simulink library "dsrc_transmitter"  (Simulink 8.2)
settings: Solver=ode1  StartTime=0.0  StopTime=Inf  FixedStep=0.001  RelTol=1e-3
PostLoadFcn:
  | , if any(exist('dsrtsu_mdlpostloadfcn', 'file') == [2, 3, 6]), try dsrtsu_mdlpostloadfcn('Execute', bdroot); catch fprintf('Error in PostLoadFcn (dsrtsu_mdlpostloadfcn) for model "%s":\n %s\n', bdroot, lasterr); end, end,
libraries: simulink x10, rtitttasklib x2, rtiethernetudplib x1, parse_utils x1
(part 2 of 2)

== system dsrc_transmitter/BSM Broadcast/Write TORC Data/Veh 3 Data Update ==
  BSM Data1 : Inport
  Action Port : ActionPort
  Bus Selector : BusSelector  OutputSignals=signal1 (signal 1),value (signal 2),value (signal 3),signal4 (signal 4),signal5 (signal 5),signal6 (signal 6),value (signal 7),value (signal 8),value (signal 9),value (signal 10),value (signal 11),value (signal 12),value (signal 13),value (signal 14),value (signal 15),signal16 (signal 16),signal17 (signal 17),signal18 (signal 18),signal19 (signal 19),signal20 (signal 20),signal21 (signal 21),signal22 (signal 22),signal23 (signal 23),signal24 (signal 24),signal25 (signal 25),value (signal 26),value (signal 27),signal28 (signal 28),value (signal 29),signal30 (signal 30),value (signal 31),signal32 (signal 32),signal33 (signal 33),value (signal 34),value (signal 35),signal36 (signal 36),signal37 (signal 37),signal38 (signal 38),signal39 (signal 39),signal40 (signal 40),signal41 (signal 41),signal42 (signal 42),signal43 (signal 43),signal44 (signal 44),signal45 (signal 45)
  Data Store Write1 : DataStoreWrite  DataStoreName=BSMStoreSignal  DataStoreElements=BSMStoreSignal.Veh3BSM.caccFlags_bitmask#BSMStoreSignal.Veh3BSM.setSpeed_m_s#BSMStoreSignal.Veh3BSM.throtPos_percent#BSMStoreSignal.Veh3BSM.lclPN_mm#BSMStoreSignal.Veh3BSM.lclPE_mm#BSMStoreSignal.Veh3BSM.lclPD_mm#BSMStoreSignal.Veh3BSM.roll_deg#BSMStoreSignal.Veh3BSM.pitch_deg#BSMStoreSignal.Veh3BSM.yaw_deg#BSMStoreSignal.Veh3BSM.hPosAcry_m#BSMStoreSignal.Veh3BSM.vPosAcry_m#BSMStoreSignal.Veh3BSM.frwdVel_m_s#BSMStoreSignal.Veh3BSM.rightVel_m_s#BSMStoreSignal.Veh3BSM.downVel_m_s#BSMStoreSignal.Veh3BSM.velAcc_m_s#BSMStoreSignal.Veh3BSM.frwdAcc_mm_s_s#BSMStoreSignal.Veh3BSM.rightAcc_mm_s_s#BSMStoreSignal.Veh3BSM.dwnAcc_mm_s_s#BSMStoreSignal.Veh3BSM.msgID#BSMStoreSignal.Veh3BSM.msgCnt#BSMStoreSignal.Veh3BSM.id#BSMStoreSignal.Veh3BSM.secMark_ms#BSMStoreSignal.Veh3BSM.lat_deg#BSMStoreSignal.Veh3BSM.lon_deg#BSMStoreSignal.Veh3BSM.elev_m#BSMStoreSignal.Veh3BSM.semi_major_accuracy_m#BSMStoreSignal.Veh3BSM.semi_minor_accuracy_m#BSMStoreSignal.Veh3BSM.semi_major_accuracy_orientation_deg#BSMStoreSignal.Veh3BSM.speed_m_s#BSMStoreSignal.Veh3BSM.transmission_enum#BSMStoreSignal.Veh3BSM.heading_deg#BSMStoreSignal.Veh3BSM.angle_deg#BSMStoreSignal.Veh3BSM.vertical_acceleration_g#BSMStoreSignal.Veh3BSM.lat_acceleration_m_s_s#BSMStoreSignal.Veh3BSM.long_acceleration_m_s_s#BSMStoreSignal.Veh3BSM.yaw_rate_deg_s#BSMStoreSignal.Veh3BSM.wheelBrakes_bitmask#BSMStoreSignal.Veh3BSM.wheelBrakesUnavailable#BSMStoreSignal.Veh3BSM.tractionControlState_enum#BSMStoreSignal.Veh3BSM.anti_lock_brake_status_enum#BSMStoreSignal.Veh3BSM.stability_control_status_enum#BSMStoreSignal.Veh3BSM.brake_boost_enum#BSMStoreSignal.Veh3BSM.auxiliary_brakes_status_enum#BSMStoreSignal.Veh3BSM.vehicle_height_cm#BSMStoreSignal.Veh3BSM.vehicle_width_cm
  wires:
  BSM Data1/1 -> Bus Selector/1
  Bus Selector/31 -> Data Store Write1/31  "<value (signal 31)>"
  Bus Selector/10 -> Data Store Write1/10  "<value (signal 10)>"
  Bus Selector/8 -> Data Store Write1/8  "<value (signal 8)>"
  Bus Selector/13 -> Data Store Write1/13  "<value (signal 13)>"
  Bus Selector/11 -> Data Store Write1/11  "<value (signal 11)>"
  Bus Selector/12 -> Data Store Write1/12  "<value (signal 12)>"
  Bus Selector/19 -> Data Store Write1/19  "<signal19 (signal 19)>"
  Bus Selector/20 -> Data Store Write1/20  "<signal20 (signal 20)>"
  Bus Selector/18 -> Data Store Write1/18  "<signal18 (signal 18)>"
  Bus Selector/14 -> Data Store Write1/14  "<value (signal 14)>"
  Bus Selector/22 -> Data Store Write1/22  "<signal22 (signal 22)>"
  Bus Selector/44 -> Data Store Write1/44  "<signal44 (signal 44)>"
  Bus Selector/42 -> Data Store Write1/42  "<signal42 (signal 42)>"
  Bus Selector/35 -> Data Store Write1/35  "<value (signal 35)>"
  Bus Selector/36 -> Data Store Write1/36  "<signal36 (signal 36)>"
  Bus Selector/45 -> Data Store Write1/45  "<signal45 (signal 45)>"
  Bus Selector/7 -> Data Store Write1/7  "<value (signal 7)>"
  Bus Selector/39 -> Data Store Write1/39  "<signal39 (signal 39)>"
  Bus Selector/23 -> Data Store Write1/23  "<signal23 (signal 23)>"
  Bus Selector/43 -> Data Store Write1/43  "<signal43 (signal 43)>"
  Bus Selector/28 -> Data Store Write1/28  "<signal28 (signal 28)>"
  Bus Selector/29 -> Data Store Write1/29  "<value (signal 29)>"
  Bus Selector/25 -> Data Store Write1/25  "<signal25 (signal 25)>"
  Bus Selector/30 -> Data Store Write1/30  "<signal30 (signal 30)>"
  Bus Selector/32 -> Data Store Write1/32  "<signal32 (signal 32)>"
  Bus Selector/27 -> Data Store Write1/27  "<value (signal 27)>"
  Bus Selector/26 -> Data Store Write1/26  "<value (signal 26)>"
  Bus Selector/24 -> Data Store Write1/24  "<signal24 (signal 24)>"
  Bus Selector/16 -> Data Store Write1/16  "<signal16 (signal 16)>"
  Bus Selector/33 -> Data Store Write1/33  "<signal33 (signal 33)>"
  Bus Selector/17 -> Data Store Write1/17  "<signal17 (signal 17)>"
  Bus Selector/15 -> Data Store Write1/15  "<value (signal 15)>"
  Bus Selector/41 -> Data Store Write1/41  "<signal41 (signal 41)>"
  Bus Selector/37 -> Data Store Write1/37  "<signal37 (signal 37)>"
  Bus Selector/9 -> Data Store Write1/9  "<value (signal 9)>"
  Bus Selector/3 -> Data Store Write1/3  "<value (signal 3)>"
  Bus Selector/38 -> Data Store Write1/38  "<signal38 (signal 38)>"
  Bus Selector/5 -> Data Store Write1/5  "<signal5 (signal 5)>"
  Bus Selector/4 -> Data Store Write1/4  "<signal4 (signal 4)>"
  Bus Selector/1 -> Data Store Write1/1  "<signal1 (signal 1)>"
  Bus Selector/40 -> Data Store Write1/40  "<signal40 (signal 40)>"
  Bus Selector/2 -> Data Store Write1/2  "<value (signal 2)>"
  Bus Selector/34 -> Data Store Write1/34  "<value (signal 34)>"
  Bus Selector/21 -> Data Store Write1/21  "<signal21 (signal 21)>"
  Bus Selector/6 -> Data Store Write1/6  "<signal6 (signal 6)>"

== system dsrc_transmitter/BSM Broadcast/Write TORC Data/Veh 4 Data Update ==
  BSM Data : Inport
  Action Port : ActionPort
  Bus Selector : BusSelector  OutputSignals=signal1 (signal 1),value (signal 2),value (signal 3),signal4 (signal 4),signal5 (signal 5),signal6 (signal 6),value (signal 7),value (signal 8),value (signal 9),value (signal 10),value (signal 11),value (signal 12),value (signal 13),value (signal 14),value (signal 15),signal16 (signal 16),signal17 (signal 17),signal18 (signal 18),signal19 (signal 19),signal20 (signal 20),signal21 (signal 21),signal22 (signal 22),signal23 (signal 23),signal24 (signal 24),signal25 (signal 25),value (signal 26),value (signal 27),signal28 (signal 28),value (signal 29),signal30 (signal 30),value (signal 31),signal32 (signal 32),signal33 (signal 33),value (signal 34),value (signal 35),signal36 (signal 36),signal37 (signal 37),signal38 (signal 38),signal39 (signal 39),signal40 (signal 40),signal41 (signal 41),signal42 (signal 42),signal43 (signal 43),signal44 (signal 44),signal45 (signal 45)
  Data Store Write1 : DataStoreWrite  DataStoreName=BSMStoreSignal  DataStoreElements=BSMStoreSignal.Veh4BSM.caccFlags_bitmask#BSMStoreSignal.Veh4BSM.setSpeed_m_s#BSMStoreSignal.Veh4BSM.throtPos_percent#BSMStoreSignal.Veh4BSM.lclPN_mm#BSMStoreSignal.Veh4BSM.lclPE_mm#BSMStoreSignal.Veh4BSM.lclPD_mm#BSMStoreSignal.Veh4BSM.roll_deg#BSMStoreSignal.Veh4BSM.pitch_deg#BSMStoreSignal.Veh4BSM.yaw_deg#BSMStoreSignal.Veh4BSM.hPosAcry_m#BSMStoreSignal.Veh4BSM.vPosAcry_m#BSMStoreSignal.Veh4BSM.frwdVel_m_s#BSMStoreSignal.Veh4BSM.rightVel_m_s#BSMStoreSignal.Veh4BSM.downVel_m_s#BSMStoreSignal.Veh4BSM.velAcc_m_s#BSMStoreSignal.Veh4BSM.frwdAcc_mm_s_s#BSMStoreSignal.Veh4BSM.rightAcc_mm_s_s#BSMStoreSignal.Veh4BSM.dwnAcc_mm_s_s#BSMStoreSignal.Veh4BSM.msgID#BSMStoreSignal.Veh4BSM.msgCnt#BSMStoreSignal.Veh4BSM.id#BSMStoreSignal.Veh4BSM.secMark_ms#BSMStoreSignal.Veh4BSM.lat_deg#BSMStoreSignal.Veh4BSM.lon_deg#BSMStoreSignal.Veh4BSM.elev_m#BSMStoreSignal.Veh4BSM.semi_major_accuracy_m#BSMStoreSignal.Veh4BSM.semi_minor_accuracy_m#BSMStoreSignal.Veh4BSM.semi_major_accuracy_orientation_deg#BSMStoreSignal.Veh4BSM.speed_m_s#BSMStoreSignal.Veh4BSM.transmission_enum#BSMStoreSignal.Veh4BSM.heading_deg#BSMStoreSignal.Veh4BSM.angle_deg#BSMStoreSignal.Veh4BSM.vertical_acceleration_g#BSMStoreSignal.Veh4BSM.lat_acceleration_m_s_s#BSMStoreSignal.Veh4BSM.long_acceleration_m_s_s#BSMStoreSignal.Veh4BSM.yaw_rate_deg_s#BSMStoreSignal.Veh4BSM.wheelBrakes_bitmask#BSMStoreSignal.Veh4BSM.wheelBrakesUnavailable#BSMStoreSignal.Veh4BSM.tractionControlState_enum#BSMStoreSignal.Veh4BSM.anti_lock_brake_status_enum#BSMStoreSignal.Veh4BSM.stability_control_status_enum#BSMStoreSignal.Veh4BSM.brake_boost_enum#BSMStoreSignal.Veh4BSM.auxiliary_brakes_status_enum#BSMStoreSignal.Veh4BSM.vehicle_height_cm#BSMStoreSignal.Veh4BSM.vehicle_width_cm
  wires:
  BSM Data/1 -> Bus Selector/1
  Bus Selector/31 -> Data Store Write1/31  "<value (signal 31)>"
  Bus Selector/10 -> Data Store Write1/10  "<value (signal 10)>"
  Bus Selector/8 -> Data Store Write1/8  "<value (signal 8)>"
  Bus Selector/13 -> Data Store Write1/13  "<value (signal 13)>"
  Bus Selector/11 -> Data Store Write1/11  "<value (signal 11)>"
  Bus Selector/12 -> Data Store Write1/12  "<value (signal 12)>"
  Bus Selector/19 -> Data Store Write1/19  "<signal19 (signal 19)>"
  Bus Selector/20 -> Data Store Write1/20  "<signal20 (signal 20)>"
  Bus Selector/18 -> Data Store Write1/18  "<signal18 (signal 18)>"
  Bus Selector/14 -> Data Store Write1/14  "<value (signal 14)>"
  Bus Selector/22 -> Data Store Write1/22  "<signal22 (signal 22)>"
  Bus Selector/44 -> Data Store Write1/44  "<signal44 (signal 44)>"
  Bus Selector/42 -> Data Store Write1/42  "<signal42 (signal 42)>"
  Bus Selector/35 -> Data Store Write1/35  "<value (signal 35)>"
  Bus Selector/36 -> Data Store Write1/36  "<signal36 (signal 36)>"
  Bus Selector/45 -> Data Store Write1/45  "<signal45 (signal 45)>"
  Bus Selector/7 -> Data Store Write1/7  "<value (signal 7)>"
  Bus Selector/39 -> Data Store Write1/39  "<signal39 (signal 39)>"
  Bus Selector/23 -> Data Store Write1/23  "<signal23 (signal 23)>"
  Bus Selector/43 -> Data Store Write1/43  "<signal43 (signal 43)>"
  Bus Selector/28 -> Data Store Write1/28  "<signal28 (signal 28)>"
  Bus Selector/29 -> Data Store Write1/29  "<value (signal 29)>"
  Bus Selector/25 -> Data Store Write1/25  "<signal25 (signal 25)>"
  Bus Selector/30 -> Data Store Write1/30  "<signal30 (signal 30)>"
  Bus Selector/32 -> Data Store Write1/32  "<signal32 (signal 32)>"
  Bus Selector/27 -> Data Store Write1/27  "<value (signal 27)>"
  Bus Selector/26 -> Data Store Write1/26  "<value (signal 26)>"
  Bus Selector/24 -> Data Store Write1/24  "<signal24 (signal 24)>"
  Bus Selector/16 -> Data Store Write1/16  "<signal16 (signal 16)>"
  Bus Selector/33 -> Data Store Write1/33  "<signal33 (signal 33)>"
  Bus Selector/17 -> Data Store Write1/17  "<signal17 (signal 17)>"
  Bus Selector/15 -> Data Store Write1/15  "<value (signal 15)>"
  Bus Selector/41 -> Data Store Write1/41  "<signal41 (signal 41)>"
  Bus Selector/37 -> Data Store Write1/37  "<signal37 (signal 37)>"
  Bus Selector/9 -> Data Store Write1/9  "<value (signal 9)>"
  Bus Selector/3 -> Data Store Write1/3  "<value (signal 3)>"
  Bus Selector/38 -> Data Store Write1/38  "<signal38 (signal 38)>"
  Bus Selector/5 -> Data Store Write1/5  "<signal5 (signal 5)>"
  Bus Selector/4 -> Data Store Write1/4  "<signal4 (signal 4)>"
  Bus Selector/1 -> Data Store Write1/1  "<signal1 (signal 1)>"
  Bus Selector/40 -> Data Store Write1/40  "<signal40 (signal 40)>"
  Bus Selector/2 -> Data Store Write1/2  "<value (signal 2)>"
  Bus Selector/34 -> Data Store Write1/34  "<value (signal 34)>"
  Bus Selector/21 -> Data Store Write1/21  "<signal21 (signal 21)>"
  Bus Selector/6 -> Data Store Write1/6  "<signal6 (signal 6)>"

== system dsrc_transmitter/BSM Broadcast/Write TORC Data/Veh 5 Data Update ==
  BSM Data : Inport
  Action Port : ActionPort
  Bus Selector : BusSelector  OutputSignals=signal1 (signal 1),value (signal 2),value (signal 3),signal4 (signal 4),signal5 (signal 5),signal6 (signal 6),value (signal 7),value (signal 8),value (signal 9),value (signal 10),value (signal 11),value (signal 12),value (signal 13),value (signal 14),value (signal 15),signal16 (signal 16),signal17 (signal 17),signal18 (signal 18),signal19 (signal 19),signal20 (signal 20),signal21 (signal 21),signal22 (signal 22),signal23 (signal 23),signal24 (signal 24),signal25 (signal 25),value (signal 26),value (signal 27),signal28 (signal 28),value (signal 29),signal30 (signal 30),value (signal 31),signal32 (signal 32),signal33 (signal 33),value (signal 34),value (signal 35),signal36 (signal 36),signal37 (signal 37),signal38 (signal 38),signal39 (signal 39),signal40 (signal 40),signal41 (signal 41),signal42 (signal 42),signal43 (signal 43),signal44 (signal 44),signal45 (signal 45)
  Data Store Write1 : DataStoreWrite  DataStoreName=BSMStoreSignal  DataStoreElements=BSMStoreSignal.Veh5BSM.caccFlags_bitmask#BSMStoreSignal.Veh5BSM.setSpeed_m_s#BSMStoreSignal.Veh5BSM.throtPos_percent#BSMStoreSignal.Veh5BSM.lclPN_mm#BSMStoreSignal.Veh5BSM.lclPE_mm#BSMStoreSignal.Veh5BSM.lclPD_mm#BSMStoreSignal.Veh5BSM.roll_deg#BSMStoreSignal.Veh5BSM.pitch_deg#BSMStoreSignal.Veh5BSM.yaw_deg#BSMStoreSignal.Veh5BSM.hPosAcry_m#BSMStoreSignal.Veh5BSM.vPosAcry_m#BSMStoreSignal.Veh5BSM.frwdVel_m_s#BSMStoreSignal.Veh5BSM.rightVel_m_s#BSMStoreSignal.Veh5BSM.downVel_m_s#BSMStoreSignal.Veh5BSM.velAcc_m_s#BSMStoreSignal.Veh5BSM.frwdAcc_mm_s_s#BSMStoreSignal.Veh5BSM.rightAcc_mm_s_s#BSMStoreSignal.Veh5BSM.dwnAcc_mm_s_s#BSMStoreSignal.Veh5BSM.msgID#BSMStoreSignal.Veh5BSM.msgCnt#BSMStoreSignal.Veh5BSM.id#BSMStoreSignal.Veh5BSM.secMark_ms#BSMStoreSignal.Veh5BSM.lat_deg#BSMStoreSignal.Veh5BSM.lon_deg#BSMStoreSignal.Veh5BSM.elev_m#BSMStoreSignal.Veh5BSM.semi_major_accuracy_m#BSMStoreSignal.Veh5BSM.semi_minor_accuracy_m#BSMStoreSignal.Veh5BSM.semi_major_accuracy_orientation_deg#BSMStoreSignal.Veh5BSM.speed_m_s#BSMStoreSignal.Veh5BSM.transmission_enum#BSMStoreSignal.Veh5BSM.heading_deg#BSMStoreSignal.Veh5BSM.angle_deg#BSMStoreSignal.Veh5BSM.vertical_acceleration_g#BSMStoreSignal.Veh5BSM.lat_acceleration_m_s_s#BSMStoreSignal.Veh5BSM.long_acceleration_m_s_s#BSMStoreSignal.Veh5BSM.yaw_rate_deg_s#BSMStoreSignal.Veh5BSM.wheelBrakes_bitmask#BSMStoreSignal.Veh5BSM.wheelBrakesUnavailable#BSMStoreSignal.Veh5BSM.tractionControlState_enum#BSMStoreSignal.Veh5BSM.anti_lock_brake_status_enum#BSMStoreSignal.Veh5BSM.stability_control_status_enum#BSMStoreSignal.Veh5BSM.brake_boost_enum#BSMStoreSignal.Veh5BSM.auxiliary_brakes_status_enum#BSMStoreSignal.Veh5BSM.vehicle_height_cm#BSMStoreSignal.Veh5BSM.vehicle_width_cm
  wires:
  BSM Data/1 -> Bus Selector/1
  Bus Selector/31 -> Data Store Write1/31  "<value (signal 31)>"
  Bus Selector/10 -> Data Store Write1/10  "<value (signal 10)>"
  Bus Selector/8 -> Data Store Write1/8  "<value (signal 8)>"
  Bus Selector/13 -> Data Store Write1/13  "<value (signal 13)>"
  Bus Selector/11 -> Data Store Write1/11  "<value (signal 11)>"
  Bus Selector/12 -> Data Store Write1/12  "<value (signal 12)>"
  Bus Selector/19 -> Data Store Write1/19  "<signal19 (signal 19)>"
  Bus Selector/20 -> Data Store Write1/20  "<signal20 (signal 20)>"
  Bus Selector/18 -> Data Store Write1/18  "<signal18 (signal 18)>"
  Bus Selector/14 -> Data Store Write1/14  "<value (signal 14)>"
  Bus Selector/22 -> Data Store Write1/22  "<signal22 (signal 22)>"
  Bus Selector/44 -> Data Store Write1/44  "<signal44 (signal 44)>"
  Bus Selector/42 -> Data Store Write1/42  "<signal42 (signal 42)>"
  Bus Selector/35 -> Data Store Write1/35  "<value (signal 35)>"
  Bus Selector/36 -> Data Store Write1/36  "<signal36 (signal 36)>"
  Bus Selector/45 -> Data Store Write1/45  "<signal45 (signal 45)>"
  Bus Selector/7 -> Data Store Write1/7  "<value (signal 7)>"
  Bus Selector/39 -> Data Store Write1/39  "<signal39 (signal 39)>"
  Bus Selector/23 -> Data Store Write1/23  "<signal23 (signal 23)>"
  Bus Selector/43 -> Data Store Write1/43  "<signal43 (signal 43)>"
  Bus Selector/28 -> Data Store Write1/28  "<signal28 (signal 28)>"
  Bus Selector/29 -> Data Store Write1/29  "<value (signal 29)>"
  Bus Selector/25 -> Data Store Write1/25  "<signal25 (signal 25)>"
  Bus Selector/30 -> Data Store Write1/30  "<signal30 (signal 30)>"
  Bus Selector/32 -> Data Store Write1/32  "<signal32 (signal 32)>"
  Bus Selector/27 -> Data Store Write1/27  "<value (signal 27)>"
  Bus Selector/26 -> Data Store Write1/26  "<value (signal 26)>"
  Bus Selector/24 -> Data Store Write1/24  "<signal24 (signal 24)>"
  Bus Selector/16 -> Data Store Write1/16  "<signal16 (signal 16)>"
  Bus Selector/33 -> Data Store Write1/33  "<signal33 (signal 33)>"
  Bus Selector/17 -> Data Store Write1/17  "<signal17 (signal 17)>"
  Bus Selector/15 -> Data Store Write1/15  "<value (signal 15)>"
  Bus Selector/41 -> Data Store Write1/41  "<signal41 (signal 41)>"
  Bus Selector/37 -> Data Store Write1/37  "<signal37 (signal 37)>"
  Bus Selector/9 -> Data Store Write1/9  "<value (signal 9)>"
  Bus Selector/3 -> Data Store Write1/3  "<value (signal 3)>"
  Bus Selector/38 -> Data Store Write1/38  "<signal38 (signal 38)>"
  Bus Selector/5 -> Data Store Write1/5  "<signal5 (signal 5)>"
  Bus Selector/4 -> Data Store Write1/4  "<signal4 (signal 4)>"
  Bus Selector/1 -> Data Store Write1/1  "<signal1 (signal 1)>"
  Bus Selector/40 -> Data Store Write1/40  "<signal40 (signal 40)>"
  Bus Selector/2 -> Data Store Write1/2  "<value (signal 2)>"
  Bus Selector/34 -> Data Store Write1/34  "<value (signal 34)>"
  Bus Selector/21 -> Data Store Write1/21  "<signal21 (signal 21)>"
  Bus Selector/6 -> Data Store Write1/6  "<signal6 (signal 6)>"

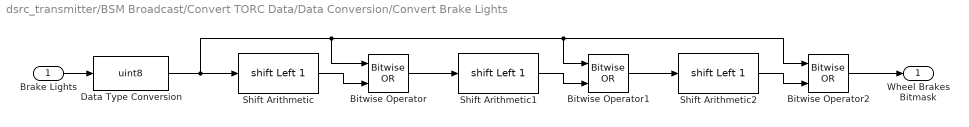
== system dsrc_transmitter/BSM Broadcast/Convert TORC Data/Data Conversion/Convert Brake Lights ==
  Brake Lights : Inport
  Bitwise Operator : simulink/Logic and Bit Operations/Bitwise Operator  logicop=OR  UseBitMask=off  NumInputPorts=2  BitMask=bin2dec('11011001')  BitMaskRealWorld=Stored Integer
  Bitwise Operator1 : simulink/Logic and Bit Operations/Bitwise Operator  logicop=OR  UseBitMask=off  NumInputPorts=2  BitMask=bin2dec('11011001')  BitMaskRealWorld=Stored Integer
  Bitwise Operator2 : simulink/Logic and Bit Operations/Bitwise Operator  logicop=OR  UseBitMask=off  NumInputPorts=2  BitMask=bin2dec('11011001')  BitMaskRealWorld=Stored Integer
  Data Type Conversion : DataTypeConversion  OutDataTypeStr=uint8
  Shift Arithmetic : ArithShift  BitShiftNumber=1  BitShiftDirection=Left
  Shift Arithmetic1 : ArithShift  BitShiftNumber=1  BitShiftDirection=Left
  Shift Arithmetic2 : ArithShift  BitShiftNumber=1  BitShiftDirection=Left
  Wheel Brakes Bitmask : Outport
  wires:
  Brake Lights/1 -> Data Type Conversion/1
  Data Type Conversion/1 -> Bitwise Operator2/1, Bitwise Operator1/1, Bitwise Operator/1, Shift Arithmetic/1
  Shift Arithmetic/1 -> Bitwise Operator/2
  Bitwise Operator/1 -> Shift Arithmetic1/1
  Shift Arithmetic1/1 -> Bitwise Operator1/2
  Bitwise Operator1/1 -> Shift Arithmetic2/1
  Shift Arithmetic2/1 -> Bitwise Operator2/2
  Bitwise Operator2/1 -> Wheel Brakes Bitmask/1

== system dsrc_transmitter/BSM Broadcast/Convert TORC Data/Data Conversion/Convert Down Acc ==
  Down Acc : Inport
  Constant : Constant  Value=1000  OutDataTypeStr=Inherit: Inherit via back propagation
  Data Type Conversion : DataTypeConversion
  Product : Product
  Down Acc mm/s/s : Outport
  wires:
  Down Acc/1 -> Product/1
  Constant/1 -> Product/2
  Data Type Conversion/1 -> Down Acc mm/s/s/1
  Product/1 -> Data Type Conversion/1

== system dsrc_transmitter/BSM Broadcast/Convert TORC Data/Data Conversion/Convert Down Acceleration ==
  Down Acc : Inport
  Constant : Constant  Value=-9.81  OutDataTypeStr=single
  Divide : Product  Inputs=*/
  g : Outport
  wires:
  Down Acc/1 -> Divide/1
  Constant/1 -> Divide/2
  Divide/1 -> g/1

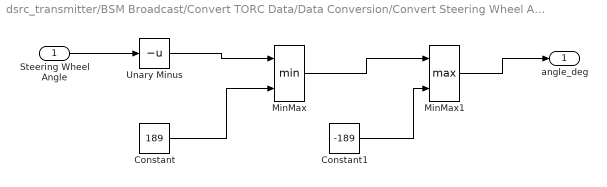
== system dsrc_transmitter/BSM Broadcast/Convert TORC Data/Data Conversion/Convert Steering Wheel Angle ==
  Steering Wheel Angle : Inport
  Constant : Constant  Value=189  OutDataTypeStr=single
  Constant1 : Constant  Value=-189  OutDataTypeStr=single
  MinMax : MinMax  Inputs=2
  MinMax1 : MinMax  Function=max  Inputs=2
  Unary Minus : UnaryMinus
  angle_deg : Outport
  wires:
  Steering Wheel Angle/1 -> Unary Minus/1
  Unary Minus/1 -> MinMax/1
  Constant/1 -> MinMax/2
  MinMax/1 -> MinMax1/1
  Constant1/1 -> MinMax1/2
  MinMax1/1 -> angle_deg/1

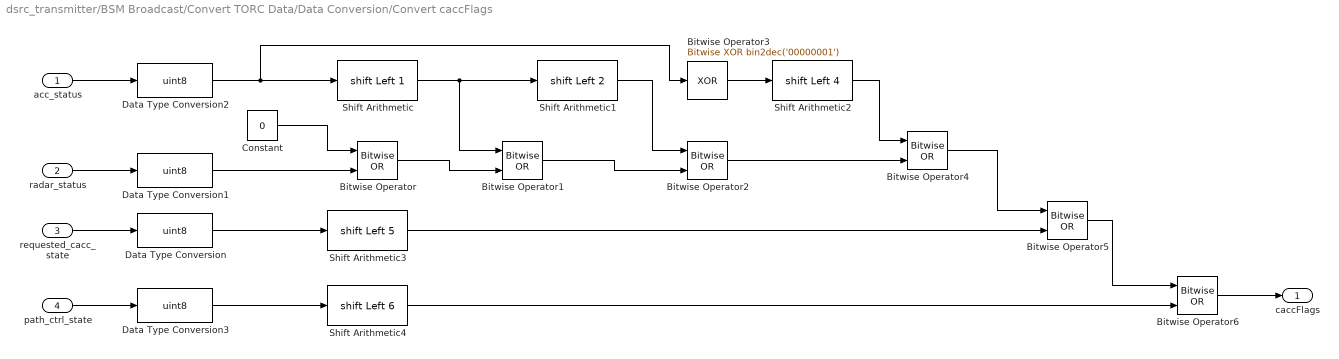
== system dsrc_transmitter/BSM Broadcast/Convert TORC Data/Data Conversion/Convert caccFlags ==
  acc_status : Inport
  radar_status : Inport  Port=2
  requested_cacc_state : Inport  Port=3
  path_ctrl_state : Inport  Port=4
  Bitwise Operator{,1..2,4..6} (6 alike) : simulink/Logic and Bit Operations/Bitwise Operator  logicop=OR  UseBitMask=off  NumInputPorts=2  BitMask=bin2dec('11011001')  BitMaskRealWorld=Stored Integer
  Bitwise Operator3 : simulink/Logic and Bit Operations/Bitwise Operator  logicop=XOR  UseBitMask=on  BitMask=bin2dec('00000001')  BitMaskRealWorld=Stored Integer
  Constant : Constant  Value=0  OutDataTypeStr=uint8
  Data Type Conversion{,1..3} (4 alike) : DataTypeConversion  OutDataTypeStr=uint8
  Shift Arithmetic : ArithShift  BitShiftNumber=1  BitShiftDirection=Left
  Shift Arithmetic1 : ArithShift  BitShiftNumber=2  BitShiftDirection=Left
  Shift Arithmetic2 : ArithShift  BitShiftNumber=4  BitShiftDirection=Left
  Shift Arithmetic3 : ArithShift  BitShiftNumber=5  BitShiftDirection=Left
  Shift Arithmetic4 : ArithShift  BitShiftNumber=6  BitShiftDirection=Left
  caccFlags : Outport
  wires:
  radar_status/1 -> Data Type Conversion1/1
  Constant/1 -> Bitwise Operator/1
  acc_status/1 -> Data Type Conversion2/1
  Shift Arithmetic/1 -> Shift Arithmetic1/1, Bitwise Operator1/1
  Bitwise Operator/1 -> Bitwise Operator1/2
  Bitwise Operator1/1 -> Bitwise Operator2/2
  Shift Arithmetic1/1 -> Bitwise Operator2/1
  Bitwise Operator3/1 -> Shift Arithmetic2/1
  Shift Arithmetic2/1 -> Bitwise Operator4/1
  Bitwise Operator2/1 -> Bitwise Operator4/2
  requested_cacc_state/1 -> Data Type Conversion/1
  Shift Arithmetic3/1 -> Bitwise Operator5/2
  Bitwise Operator4/1 -> Bitwise Operator5/1
  Data Type Conversion/1 -> Shift Arithmetic3/1
  Data Type Conversion1/1 -> Bitwise Operator/2
  Data Type Conversion2/1 -> Bitwise Operator3/1, Shift Arithmetic/1
  path_ctrl_state/1 -> Data Type Conversion3/1
  Data Type Conversion3/1 -> Shift Arithmetic4/1
  Shift Arithmetic4/1 -> Bitwise Operator6/2
  Bitwise Operator5/1 -> Bitwise Operator6/1
  Bitwise Operator6/1 -> caccFlags/1

== system dsrc_transmitter/BSM Broadcast/Convert TORC Data/Data Conversion/Convert fwrdAcc ==
  fwrdAcc_m_s_s : Inport
  Constant : Constant  Value=1000
  Data Type Conversion : DataTypeConversion  OutDataTypeStr=int16
  Product : Product
  fwrdAcc_mm_s_s : Outport
  wires:
  fwrdAcc_m_s_s/1 -> Product/1
  Data Type Conversion/1 -> fwrdAcc_mm_s_s/1
  Product/1 -> Data Type Conversion/1
  Constant/1 -> Product/2

== system dsrc_transmitter/BSM Broadcast/Convert TORC Data/Data Conversion/Convert rightAcc ==
  rightAcc_m_s_s : Inport
  Constant : Constant  Value=1000
  Data Type Conversion : DataTypeConversion  OutDataTypeStr=int16
  Product : Product
  rightAcc_mm_s_s : Outport
  wires:
  rightAcc_m_s_s/1 -> Product/1
  Data Type Conversion/1 -> rightAcc_mm_s_s/1
  Product/1 -> Data Type Conversion/1
  Constant/1 -> Product/2

== system dsrc_transmitter/BSM Broadcast/Convert TORC Data/Data Conversion/Convert utcTime ==
  utcTime : Inport
  Constant : Constant  Value=60000
  Constant1 : Constant  Value=1000
  Data Type Conversion : DataTypeConversion  RndMeth=Round
  Math Function : Math  Operator=mod  SaturateOnIntegerOverflow=on
  Product : Product
  secMark : Outport
  wires:
  Constant/1 -> Math Function/2
  Math Function/1 -> Data Type Conversion/1
  Data Type Conversion/1 -> secMark/1
  utcTime/1 -> Product/1
  Product/1 -> Math Function/1
  Constant1/1 -> Product/2

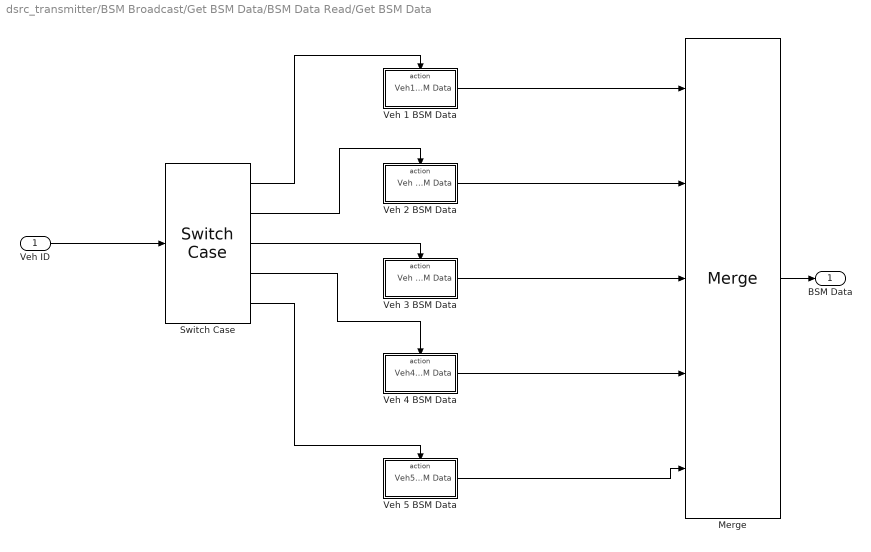
== system dsrc_transmitter/BSM Broadcast/Get BSM Data/BSM Data Read/Get BSM Data ==
  Veh ID : Inport
  Merge : Merge  Inputs=5
  Switch Case : SwitchCase  CaseConditions={96, 97, 98, 99, 100}  ShowDefaultCase=off
  Veh 1 BSM Data : Subsystem  TreatAsAtomicUnit=on
  Veh 2 BSM Data : Subsystem  TreatAsAtomicUnit=on
  Veh 3 BSM Data : Subsystem  TreatAsAtomicUnit=on
  Veh 4 BSM Data : Subsystem  TreatAsAtomicUnit=on
  Veh 5 BSM Data : Subsystem  TreatAsAtomicUnit=on
  BSM Data : Outport
  wires:
  Veh ID/1 -> Switch Case/1
  Switch Case/2 -> Veh 2 BSM Data/Action
  Switch Case/5 -> Veh 5 BSM Data/Action
  Switch Case/1 -> Veh 1 BSM Data/Action
  Switch Case/3 -> Veh 3 BSM Data/Action
  Veh 2 BSM Data/1(Veh 2 BSM Data) -> Merge/2
  Switch Case/4 -> Veh 4 BSM Data/Action
  Veh 1 BSM Data/1(Veh1 BSM Data) -> Merge/1
  Merge/1 -> BSM Data/1
  Veh 3 BSM Data/1(Veh 3 BSM Data) -> Merge/3
  Veh 5 BSM Data/1(Veh5 BSM Data) -> Merge/5
  Veh 4 BSM Data/1(Veh4 BSM Data) -> Merge/4

== system dsrc_transmitter/BSM Broadcast/Get BSM Data/BSM Data Read/Get BSM Data/Veh 1 BSM Data ==
  Action Port : ActionPort  ActionType=case
  Data Store Read : DataStoreRead  DataStoreName=BSMStoreSignal  DataStoreElements=BSMStoreSignal.Veh1BSM
  Veh1 BSM Data : Outport
  wires:
  Data Store Read/1 -> Veh1 BSM Data/1

== system dsrc_transmitter/BSM Broadcast/Get BSM Data/BSM Data Read/Get BSM Data/Veh 2 BSM Data ==
  Action Port : ActionPort  ActionType=case
  Data Store Read : DataStoreRead  DataStoreName=BSMStoreSignal  DataStoreElements=BSMStoreSignal.Veh2BSM
  Veh 2 BSM Data : Outport
  wires:
  Data Store Read/1 -> Veh 2 BSM Data/1

== system dsrc_transmitter/BSM Broadcast/Get BSM Data/BSM Data Read/Get BSM Data/Veh 3 BSM Data ==
  Action Port : ActionPort  ActionType=case
  Data Store Read : DataStoreRead  DataStoreName=BSMStoreSignal  DataStoreElements=BSMStoreSignal.Veh3BSM
  Veh 3 BSM Data : Outport
  wires:
  Data Store Read/1 -> Veh 3 BSM Data/1

== system dsrc_transmitter/BSM Broadcast/Get BSM Data/BSM Data Read/Get BSM Data/Veh 4 BSM Data ==
  Action Port : ActionPort  ActionType=case
  Data Store Read : DataStoreRead  DataStoreName=BSMStoreSignal  DataStoreElements=BSMStoreSignal.Veh4BSM
  Veh4 BSM Data : Outport
  wires:
  Data Store Read/1 -> Veh4 BSM Data/1

== system dsrc_transmitter/BSM Broadcast/Get BSM Data/BSM Data Read/Get BSM Data/Veh 5 BSM Data ==
  Action Port : ActionPort  ActionType=case
  Data Store Read : DataStoreRead  DataStoreName=BSMStoreSignal  DataStoreElements=BSMStoreSignal.Veh5BSM
  Veh5 BSM Data : Outport
  wires:
  Data Store Read/1 -> Veh5 BSM Data/1
